simulink model "electrical_model"  (R2026a)
settings: Solver=VariableStepAuto  StopTime=300
undefined symbols (not defined in the file): engine
settings Model: Creator=GOD  LastModifiedBy=GOD

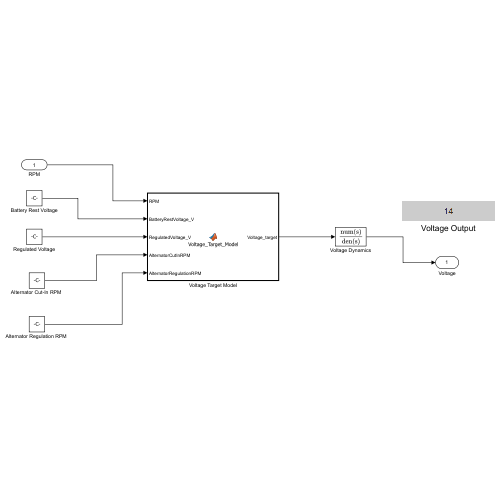
[thumbnail: Simulink's stored preview of the top-level diagram]
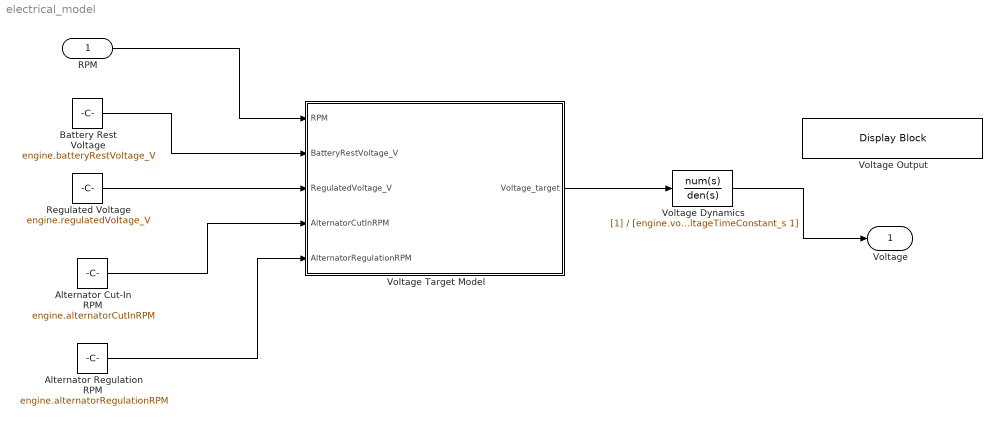
== system electrical_model ==
  RPM : Inport
  "Alternator Cut-In RPM " : Constant  Value=engine.alternatorCutInRPM
  "Alternator Regulation RPM " : Constant  Value=engine.alternatorRegulationRPM
  Battery Rest Voltage : Constant  Value=engine.batteryRestVoltage_V
  Regulated Voltage : Constant  Value=engine.regulatedVoltage_V
  Voltage Dynamics : TransferFcn  Denominator=[engine.voltageTimeConstant_s 1]
  Voltage Output : DisplayBlock  LabelPosition=Hide  Transparency=1  GridColor=[0.502, 0.502, 0.502]
  Voltage Target Model : MATLAB Function  TreatAsAtomicUnit=on
  Voltage : Outport
  wires:
  Battery Rest Voltage/1 -> Voltage Target Model/2(BatteryRestVoltage_V)
  Regulated Voltage/1 -> Voltage Target Model/3(RegulatedVoltage_V)
  "Alternator Cut-In RPM "/1 -> Voltage Target Model/4(AlternatorCutInRPM)
  "Alternator Regulation RPM "/1 -> Voltage Target Model/5(AlternatorRegulationRPM)
  Voltage Target Model/1(Voltage_target) -> Voltage Dynamics/1
  Voltage Dynamics/1 -> Voltage/1
  RPM/1 -> Voltage Target Model/1(RPM)

== matlab function electrical_model/Voltage Target Model ==
  data: RPM input; Voltage_target output; BatteryRestVoltage_V input; RegulatedVoltage_V input; AlternatorCutInRPM input; AlternatorRegulationRPM input
function Voltage_target = Voltage_Target_Model(RPM, BatteryRestVoltage_V, ...
    RegulatedVoltage_V, AlternatorCutInRPM, ...
    AlternatorRegulationRPM)
% Engineering-assumption alternator/battery voltage model.
% Below cut-in RPM the alternator isn't generating -- system runs on
% battery rest voltage. Above regulation RPM the voltage regulator
% holds a steady charging voltage. In between, voltage ramps linearly.
if RPM <= AlternatorCutInRPM
    Voltage_target = BatteryRestVoltage_V;
elseif RPM >= AlternatorRegulationRPM
    Voltage_target = RegulatedVoltage_V;
else
    frac = (RPM - AlternatorCutInRPM) / (AlternatorRegulationRPM - AlternatorCutInRPM);
    Voltage_target = BatteryRestVoltage_V + (RegulatedVoltage_V - BatteryRestVoltage_V) * frac;
end
end
